simulink model "Project_CRDI"  (R2019a)
settings: Solver=FixedStepAuto  StartTime=0.0  StopTime=10.0  FixedStep=1  RelTol=1e-3
settings Model: Creator=Akshay  LastModifiedBy=Akshay

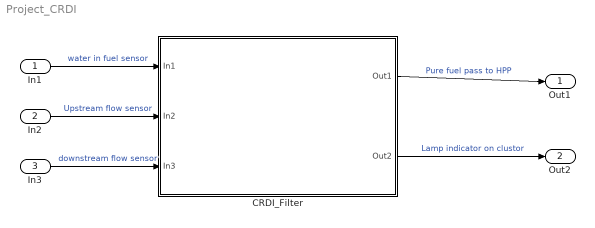
== system Project_CRDI ==
  In1 : Inport
  In2 : Inport  Port=2
  In3 : Inport  Port=3
  CRDI_Filter : Subsystem
  Out1 : Outport
  Out2 : Outport  Port=2
  wires:
  CRDI_Filter/1(Out1) -> Out1/1  "Pure fuel pass to HPP"
  CRDI_Filter/2(Out2) -> Out2/1  "Lamp indicator on clustor"
  In1/1 -> CRDI_Filter/1(In1)  "water in fuel sensor"
  In3/1 -> CRDI_Filter/3(In3)  "downstream flow sensor"
  In2/1 -> CRDI_Filter/2(In2)  "Upstream flow sensor"

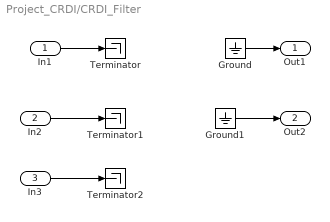
== system Project_CRDI/CRDI_Filter ==
  In1 : Inport
  In2 : Inport  Port=2
  In3 : Inport  Port=3
  Ground : Ground
  Ground1 : Ground
  Terminator : Terminator
  Terminator1 : Terminator
  Terminator2 : Terminator
  Out1 : Outport
  Out2 : Outport  Port=2
  wires:
  In1/1 -> Terminator/1
  In2/1 -> Terminator1/1
  Ground/1 -> Out1/1
  Ground1/1 -> Out2/1
  In3/1 -> Terminator2/1
